simulink model "CommandeMoteurBF"  (R2021b)
settings: Solver=VariableStepAuto  StartTime=0.0  StopTime=10.0  RelTol=1e-3
libraries: arduinolib x2
settings Model: Creator=xavier.pessoles2  LastModifiedBy=xavier.pessoles2

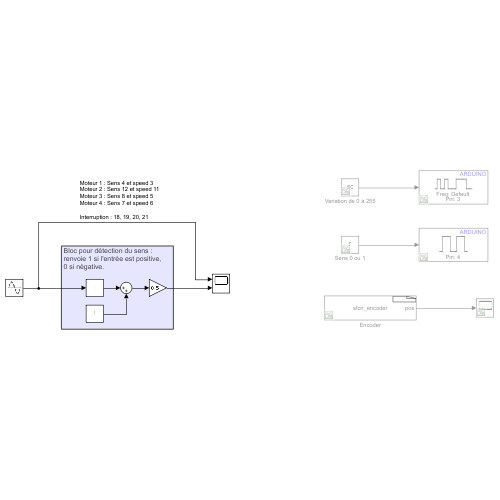
[thumbnail: Simulink's stored preview of the top-level diagram]
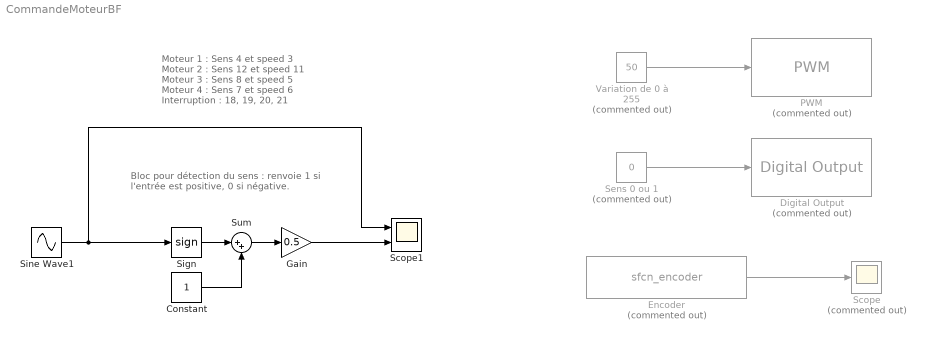
== system CommandeMoteurBF ==
  note: Bloc pour détection du sens :
      | renvoie 1 si l'entrée est positive,
      | 0 si négative.
  note: Moteur 1 : Sens 4 et speed 3
      | Moteur 2 : Sens 12 et speed 11
      | Moteur 3 : Sens 8 et speed 5
      | Moteur 4 : Sens 7 et speed 6
      |
      | Interruption : 18, 19, 20, 21
  Constant : Constant
  Digital Output : arduinolib/Digital Output  Commented=on  pinNumber=4  Direction=output  blockPlatform=arduino
  Encoder : S-Function  Commented=on  InitFcn=try, set_param(gcb,'FunctionName','sfcn_encoder'), end  FunctionName=sfcn_encoder  Parameters=uint8(0),uint8(18),uint8(19)  SFunctionModules=sfcn_encoder_wrapper  SFunctionDeploymentMode=off  EnableBusSupport=off  mask(S-Function Builder){}
      mask init:
      | val = [[.9  0.75 0.75 1 1 .9 .9 1]',[1 1 0.75 0.75 .9 .9 1 .9]'];try , sys = get_param(gcb,'SfunBuilderFcnName');if isempty(sys), sys = get_param(gcb,'FunctionName'); end,catch, sys = get_param(gcb,'FunctionName'); end
      settings: CopyFcn=set_param(gcbh,'LinkStatus','none')  PreSaveFcn=try, set_param(gcb,'FunctionName','sfcn_encoder'), end  OpenFcn=sfunctionwizard(gcbh)
      mask Display:
      | plot(val(:,1),val(:,2))
      | disp(sys)
      | port_label('output',1,'pos')
  Gain : Gain  Gain=0.5
  PWM : arduinolib/PWM  Commented=on  pinNumber=3  frequencyType=Default  desiredFrequency=490.2  achievableFrequency=490.2
  Scope : Scope  Commented=on
  Scope1 : Scope  NumInputPorts=2
  Sens 0 ou 1 : Constant  Commented=on  Value=0
  Sign : Signum
  Sine Wave1 : Sin  Amplitude=3  SampleTime=0
  Sum : Sum  Inputs=|++
  Variation de 0 à 255 : Constant  Commented=on  Value=50
  wires:
  Encoder/1 -> Scope/1
  Variation de 0 à 255/1 -> PWM/1
  Sens 0 ou 1/1 -> Digital Output/1
  Sine Wave1/1 -> Sign/1, Scope1/1
  Constant/1 -> Sum/2
  Sign/1 -> Sum/1
  Sum/1 -> Gain/1
  Gain/1 -> Scope1/2
